simulink model "PruebaSerial"  (R2022b)
settings: Solver=ode4  StartTime=0.0  StopTime=100  FixedStep=0.01  RelTol=1e-3
undefined symbols (not defined in the file or in its folder): CR, LF
libraries: instrumentseriallib x2
settings Model: Creator=lalo_  LastModifiedBy=lalo_

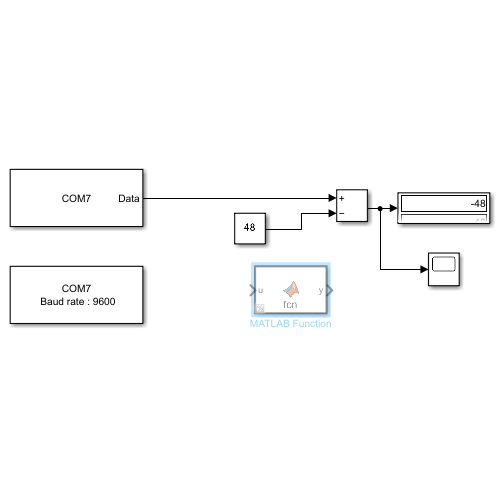
[thumbnail: Simulink's stored preview of the top-level diagram]
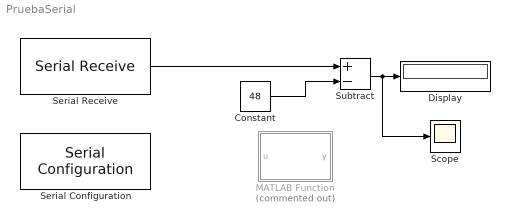
== system PruebaSerial ==
  Constant : Constant  Value=48
  Display : Display
      settings: Format=decimal (Stored Integer)
  MATLAB Function : MATLAB Function  Commented=on  TreatAsAtomicUnit=on
  Scope : Scope
  Serial Configuration : instrumentseriallib/Serial Configuration  Priority=-200000  PortSel=COM7  Port=COM7  ComPort=COM7  BaudRate=9600  DataBits=8  Parity=none  StopBits=1  ByteOrder=little-endian  FlowControl=none  Timeout=10  SimulateUsing=Interpreted execution  BlockInModel=on  aMode=1
  Serial Receive : instrumentseriallib/Serial Receive  Priority=1  PortSel=COM7  Port=COM7  ComPort=COM7  DataType=uint8  SaveDataType=uint8  ToggleHeader=off  Header=[]  ToggleTerminator=on  Terminator=CR/LF ('\r\n')  CustomTerminator=[44]  InputFormat=Column major  ToggleDataSize=on  DataSize=[1 3]  EnableBlockingMode=on  ActionDataUnavailable=Output last received value  ActionWhenDataUnavailable=Output last received value  CustomValue=0  SampleTime=0.1  SimulateUsing=Interpreted execution  BlockInModel=on  aMode=1
  Subtract : Sum  Inputs=+-
  wires:
  Serial Receive/1 -> Subtract/1
  Constant/1 -> Subtract/2
  Subtract/1 -> Scope/1, Display/1

== matlab function PruebaSerial/MATLAB Function ==
  data: u input; y output
function y = fcn(u)

y = u;
